simulink model "StateSpaceControllerRobust"  (R2020b)
settings: Solver=ode45  StartTime=0.0  StopTime=30  MaxStep=0.001  RelTol=1e-3
settings Model: Creator=umberto  LastModifiedBy=umberto

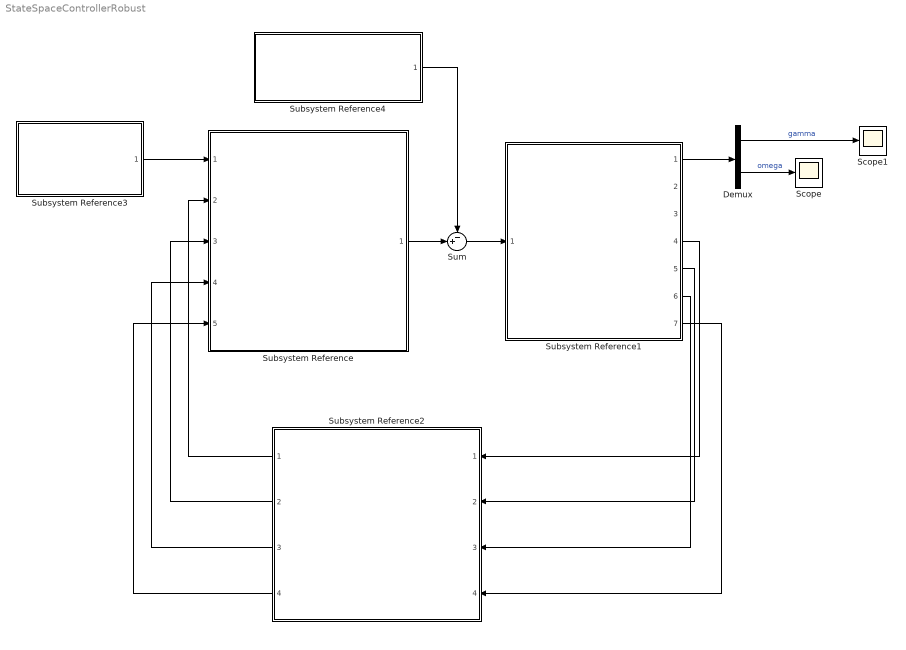
== system StateSpaceControllerRobust ==
  Demux : Demux  Outputs=2
  Scope : Scope
  Scope1 : Scope
  Subsystem Reference : Subsystem  ReferencedSubsystem=StateSpaceControllerRobust_SubSystem
  Subsystem Reference1 : Subsystem  ReferencedSubsystem=Robot_SubSystem
  Subsystem Reference2 : Subsystem  ReferencedSubsystem=SimpleStateObserver_SubSystem
  Subsystem Reference3 : Subsystem  ReferencedSubsystem=GeneratorGam_ref_SubSystem
  Subsystem Reference4 : Subsystem  ReferencedSubsystem=DisturbanceGenerator_SubSystem
  Sum : Sum  Inputs=-+|
  wires:
  Subsystem Reference1/4 -> Subsystem Reference2/1
  Subsystem Reference1/5 -> Subsystem Reference2/2
  Subsystem Reference1/6 -> Subsystem Reference2/3
  Subsystem Reference1/7 -> Subsystem Reference2/4
  Subsystem Reference2/1 -> Subsystem Reference/2
  Subsystem Reference2/2 -> Subsystem Reference/3
  Subsystem Reference2/3 -> Subsystem Reference/4
  Subsystem Reference2/4 -> Subsystem Reference/5
  Subsystem Reference1/1 -> Demux/1
  Demux/2 -> Scope/1  "omega"
  Demux/1 -> Scope1/1  "gamma"
  Subsystem Reference3/1 -> Subsystem Reference/1
  Subsystem Reference/1 -> Sum/2
  Sum/1 -> Subsystem Reference1/1
  Subsystem Reference4/1 -> Sum/1
